simulink model "ssc_refrigeration"  (R2021b)
settings: Solver=VariableStepAuto  StartTime=0.0  StopTime=4000  RelTol=1e-3  AbsTol=1e-3  EnableMultiTasking=on
PreLoadFcn:
  | load r134aPropertyTables
  | 
  | % Refrigerant:
  | initial_pressure = 0.6; % MPa
  | initial_quality = 0.05;
  | 
  | % Environment:
  | environment_temperature = 293; % K
  | natural_convection_coefficient = 20; % W/m^2/K
  | 
  | % Controller:
  | target_temperature = 277; % K
  | temperature_delta = 2; % K
  | 
  | % Compressor:
  | commanded_mass_flow = 0.004; % kg/s
  | controller_time_constant = 20; % s
  | 
  | % Expansion valve:
  | min_throat_area = 0.1; % mm^2
  | max_throat_area = 1.5; % mm^2
  | min_throat_temperature = 270; % K
  | max_throat_temperature = 250; % K
  | 
  | % Heat exchangers:
  | condenser_length = 30; % m
  | evaporator_length = 30; % m
  | fin_area = 1; % m^2
  | fin_convection_coefficient = 150; % W/m^2/K
  | 
  | % Pipes:
  | pipe_diameter = 0.01; % m
  | pipe_thickness = 0.0005; % m
  | 
  | % Refrigerator compartment:
  | interior_surface_area = 4.5; % m^2
  | exterior_surface_area = 6; % m^2
  | foam_thickness = 0.03; % m
  | 
  | % Material properties:
  | copper_density = 8940; % kg/m^3
  | copper_specific_heat = 390; % J/kg/K
  | copper_conductivity = 400; % W/m/K
  | foam_conductivity = 0.03; % W/m/K
libraries: fl_lib x44, nesl_utility x3
CloseFcn:
  | try,close(h1_ssc_refrigeration),end
  | try,close(h2_ssc_refrigeration),end
  | try,close(h3_ssc_refrigeration),end
  | try,close(h4_ssc_refrigeration),end
  | try,close(h5_ssc_refrigeration),end
  | 
  | clear h1_ssc_refrigeration h2_ssc_refrigeration h3_ssc_refrigeration h4_ssc_refrigeration h5_ssc_refrigeration
  | clear simlog_ssc_refrigeration
  | 
  | clear r134aPropertyTables
  | clear initial_pressure initial_quality
  | clear environment_temperature natural_convection_coefficient
  | clear target_temperature temperature_delta
  | clear commanded_mass_flow controller_time_constant
  | clear min_throat_area max_throat_area min_throat_temperature max_throat_temperature
  | clear condenser_length evaporator_length fin_area fin_convection_coefficient
  | clear pipe_diameter pipe_thickness
  | clear interior_surface_area exterior_surface_area foam_thickness
  | clear copper_density copper_specific_heat copper_conductivity foam_conductivity
Description:
  | Two-Phase Fluid Refrigeration
settings Model: Creator=The MathWorks, Inc.  LastModifiedBy=The MathWorks, Inc.
settings SolverCC: AutoScaleAbsTol=off  AlgebraicLoopSolver=TrustRegion
settings DataIOCC: LimitDataPoints=on  MaxDataPoints=10000  SaveFormat=Array  ReturnWorkspaceOutputs=off
settings OptimizationCC: LifeSpan=inf
settings DebuggingCC: AllowSymbolicDim=off  PregeneratedLibrarySubsystemCodeDiagnostic=none  SFUnexpectedBacktrackingDiag=warning  SFNoUnconditionalDefaultTransitionDiag=warning  SFExecutionAtInitializationDiag=none  SFMachineParentedDataDiag=warning  ArithmeticOperatorsInVariantConditions=warning
settings HardwareCC: ProdBitPerPointer=32  ProdBitPerSizeT=32  ProdBitPerPtrDiffT=32  ProdLargestAtomicFloat=None  ProdIntDivRoundTo=Undefined  ProdEndianess=Unspecified  ProdWordSize=32  ProdHWDeviceType=32-bit Generic
settings ModelReferenceCC: PropagateSignalLabelsOutOfModel=off
settings SFSimCC: SimUseLocalCustomCode=off  CustomCodeUndefinedFunction=UseInterfaceOnly
settings RTWCC: RTWUseLocalCustomCode=off
settings CodeAppCC: StateflowObjectComments=on
settings GRTTargetCC: TargetLangStandard=C89/C90 (ANSI)
settings ConfigComp: CovMetricSettings=dw  CovSaveCumulativeToWorkspaceVar=on  CovSaveSingleToWorkspaceVar=on  CovExternalEMLEnable=off  CovSFcnEnable=off
settings SimscapeCC: SimscapeLogType=all  SimscapeLogSimulationStatistics=on  SimscapeLogName=simlog_ssc_refrigeration  SimscapeLogDataHistory=10000

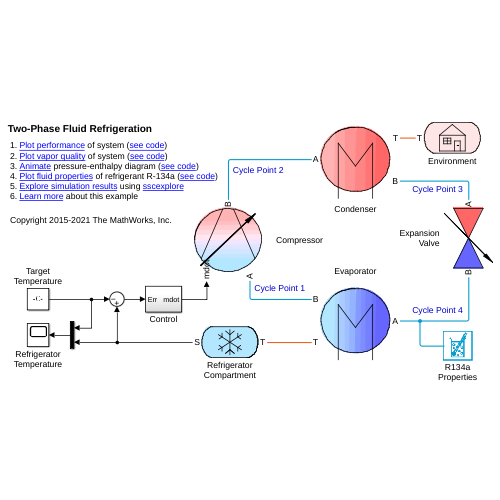
[thumbnail: Simulink's stored preview of the top-level diagram]
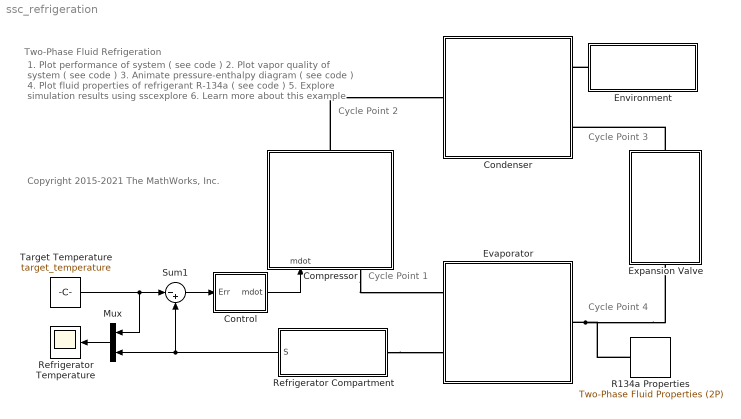
== system ssc_refrigeration ==
  note: Cycle Point 2
  note: Cycle Point 3
  note: 1. Plot performance of system ( see code )
      | 2. Plot vapor quality of system ( see code )
      | 3. Animate pressure-enthalpy diagram ( see code )
      | 4. Plot fluid properties of refrigerant R-134a ( see code )
      | 5. Explore simulation results using sscexplore
      | 6. Learn more about this example
  note: Two-Phase Fluid Refrigeration
  note: Cycle Point 4
  note: Cycle Point 1
  note: Copyright 2015-2021 The MathWorks, Inc.
  Compressor : Subsystem
      mask Display:
      | % Fading color
      | % Center to right
      | patch(sin(0.00*pi:0.05:1.10*pi),cos(0.00*pi:0.05:1.10*pi),[1;0.90;0.94]);
      | patch(sin(0.05*pi:0.05:0.95*pi),cos(0.05*pi:0.05:0.95*pi),[1;0.85;0.88]);
      | patch(sin(0.10*pi:0.05:0.90*pi),cos(0.10*pi:0.05:0.90*pi),[1;0.80;0.82]);
      | patch(sin(0.15*pi:0.05:0.85*pi),cos(0.15*pi:0.05:0.85*pi),[1;0.75;0.76]);
      | patch(sin(0.20*pi:0.05:0.80*pi),cos(0.20*pi:0.05:0.80*pi),[1;0.70;0.70]);
      | % Center to left
      | patch(sin(1.00*pi:0.05:2.00*pi),cos(1.00*pi:0.05:2.00*pi),[0.94;0.90;1]);
      | patch(sin(1.05*pi:0.05:1.95*pi),cos(1.05*pi:0.05:1.95*pi),[0.88;0.90;1]);
      | patch(sin(1.10*pi:0.05:1.90*pi),cos(1.10*pi:0.05:1.90*pi),[0.82;0.90;1]);
      | patch(sin(1.15*pi:0.05:1.85*pi),cos(1.15*pi:0.05:1.85*pi),[0.76;0.90;1]);
      | patch(sin(1.20*pi:0.05:1.80*pi),cos(1.20*pi:0.05:1.80*pi),[0.70;0.90;1]);
      | % Circle
      | plot(sin(0:0.1:2.2*pi),cos(0:0.1:2.2*pi));
      | % Angled lines
      | plot(sin([-0.6*pi/3 3.6*pi/8]),cos([-0.6*pi/3 3.6*pi/8]));
      | plot(sin([-0.6*pi/3 3.6*pi/8]),-cos([-0.6*pi/3 3.6*pi/8]));
      | plot(1.15*sin([-pi/4 3*pi/4]),1.15*cos([-pi/4 3*pi/4]));
      | % Arrow
      | patch([1.15*sin(-pi/4)+0.01;1.15*sin(3*pi/4)+0.01;1.15*sin(3*pi/4)-0.01;1.15*sin(-pi/4)-0.01],[1.15*cos(-pi/4)+0.01;1.15*cos(3*pi/4)+0.01;1.15*cos(3*pi/4)-0.01;1.15*cos(-pi/4)-0.01],[0;0;0])
      | patch([0.8*sin(3*pi/4)+0.05;1.15*sin(3*pi/4)+0.00;1.15*sin(3*pi/4)-0.00;0.8*sin(3*pi/4)-0.05],[0.8*cos(3*pi/4)+0.05;1.15*cos(3*pi/4)+0.00;1.15*cos(3*pi/4)-0.00;0.8*cos(3*pi/4)-0.05],[0;0;0])
      | % Points to set range for plotting area
      | color('white');plot(1.3,1.3);plot(-1.3,-1.3)
      | color('black');
      | 
      | port_label('LConn',1,'A');
      | port_label('RConn',1,'B');
      | port_label('input',1,'mdot');
  Condenser : Subsystem
      mask Display:
      | % Colored patches
      | % Center to right
      | patch(sin(0.0*pi:0.05:1.1*pi),cos(0.0*pi:0.05:1.1*pi),[1;0.58;0.58]);
      | patch(sin(0.1*pi:0.05:0.9*pi),cos(0.1*pi:0.05:0.9*pi),[1;0.64;0.64]);
      | patch(sin(0.2*pi:0.05:0.8*pi),cos(0.2*pi:0.05:0.8*pi),[1;0.70;0.70]);
      | % Center to left
      | patch(sin(1.0*pi:0.05:2.0*pi),cos(1.0*pi:0.05:2.0*pi),[1;0.52;0.52]);
      | patch(sin(1.1*pi:0.05:1.9*pi),cos(1.1*pi:0.05:1.9*pi),[1;0.46;0.46]);
      | patch(sin(1.2*pi:0.05:1.8*pi),cos(1.2*pi:0.05:1.8*pi),[1;0.40;0.40]);
      | % Circle
      | plot(sin(0:0.1:2.2*pi),cos(0:0.1:2.2*pi));
      | % 'M'
      | plot([0.5 0.5],[-1.2 0.5]);
      | plot([-0.5 -0.5],[-1.2 0.5]);
      | plot([0.5 0],[0.5 -0.2]);
      | plot([-0.5 0],[0.5 -0.2]);
      | % Plot points to set plot range
      | color('white');plot(1.3,1.3);plot(-1.3,-1.3)
      | color('black');
      | 
      | port_label('RConn',1,'A');
      | port_label('LConn',1,'T');
      | port_label('LConn',2,'B');
  Control : Subsystem  Tag=CustomStyle
  Environment : Subsystem
      mask Display:
      | % Colored patch
      | patch([sin(0:0.1:1*pi)*0.25+0.4 sin(pi:0.1:2*pi)*0.25-0.4],[cos(0:0.1:1*pi) cos(pi:0.1:2*pi)],[1;0.9;0.9]);
      | % Outer rounded rectangle
      | plot(sin(0:0.1:1*pi)*0.25+0.4,cos(0:0.1:1*pi));
      | plot(sin(pi:0.1:2*pi)*0.25-0.4,cos(pi:0.1:2*pi));
      | plot([-0.4 0.4],[1 1]);
      | plot([-0.4 0.4],[-1 -1]);
      | % House frame
      | plot([-0.3 -0.3],[-0.866,0.866*0.2])
      | plot([0.3 0.3],[-0.866,0.866*0.2])
      | plot([0.3 0],[0.866*0.2, 0.866])
      | plot([-0.3 0],[0.866*0.2, 0.866])
      | plot([-0.3 0.3],[-0.866 -0.866])
      | plot([-0.3 0.3],[0.866 0.866]*0.2)
      | plot([-0.2 -0.04],[0.866 0.866]*0)
      | % Window
      | plot([-0.2 -0.04],[-1 -1]*0.2)
      | plot([-0.2 -0.04],[-1 -1]*0.4)
      | plot([-0.2 -0.2],[0 -0.4])
      | plot([-0.12 -0.12],[0 -0.4])
      | plot([-0.04 -0.04],[0 -0.4])
      | % Door
      | plot([0.05 0.05],[-0.866 -0.2])
      | plot([0.18 0.18],[-0.866 -0.2])
      | plot([0.05 0.18],[-0.2 -0.2])
      | patch([0.12 0.15 0.12 0.15],[-0.5 -0.5 -0.54 -0.54],[0;0;0])
      | % Outer boundary (so plot labels are visible)
      | color('white');plot(0.8660,0.8660);plot(-0.8660,-0.8660)
      | color('black');
      | port_label('LConn',1,'T');
  Evaporator : Subsystem
      mask Display:
      | % Fading color
      | % Center to right
      | patch(sin(0.00*pi:0.05:1.10*pi),cos(0.00*pi:0.05:1.10*pi),[0.58;0.70;1]);
      | patch(sin(0.05*pi:0.05:0.95*pi),cos(0.05*pi:0.05:0.95*pi),[0.63;0.75;1]);
      | patch(sin(0.10*pi:0.05:0.90*pi),cos(0.10*pi:0.05:0.90*pi),[0.66;0.80;1]);
      | patch(sin(0.15*pi:0.05:0.85*pi),cos(0.15*pi:0.05:0.85*pi),[0.69;0.85;1]);
      | patch(sin(0.20*pi:0.05:0.80*pi),cos(0.20*pi:0.05:0.80*pi),[0.70;0.90;1]);
      | % Center to left
      | patch(sin(1.00*pi:0.05:2.00*pi),cos(1.00*pi:0.05:2.00*pi),[0.52;0.60;1]);
      | patch(sin(1.05*pi:0.05:1.95*pi),cos(1.05*pi:0.05:1.95*pi),[0.49;0.55;1]);
      | patch(sin(1.10*pi:0.05:1.90*pi),cos(1.10*pi:0.05:1.90*pi),[0.46;0.50;1]);
      | patch(sin(1.15*pi:0.05:1.85*pi),cos(1.15*pi:0.05:1.85*pi),[0.43;0.45;1]);
      | patch(sin(1.20*pi:0.05:1.80*pi),cos(1.20*pi:0.05:1.80*pi),[0.40;0.40;1]);
      | % Circle
      | plot(sin(0:0.1:2.2*pi),cos(0:0.1:2.2*pi));
      | % 'M'
      | plot([0.5 0.5],[-1.2 0.5]);
      | plot([-0.5 -0.5],[-1.2 0.5]);
      | plot([0.5 0],[0.5 -0.2]);
      | plot([-0.5 0],[0.5 -0.2]);
      | % Plot points to set plotting range
      | color('white');plot(1.3,1.3);plot(-1.3,-1.3)
      | color('black');
      | 
      | port_label('LConn',1,'A');
      | port_label('RConn',1,'B');
      | port_label('RConn',2,'T');
  Expansion Valve : Subsystem
      mask Display:
      | % Colored patches
      | patch([-1 -1 0],[0.5 -0.5 0],[1;0.4;0.4]);
      | patch([1 1 0],[0.5 -0.5 0],[0.4;0.4;1]);
      | % Valve
      | plot([1 1],[0.5 -0.5]);
      | plot([-1 -1],[0.5 -0.5]);
      | plot([-1 1],[0.5 -0.5]);
      | plot([-1 1],[-0.5 0.5]);
      | % Arrow
      | patch([1.15*sin(-pi/4-0.01);1.15*sin(-pi/4+0.01);1*sin(3*pi/4-0.01);1*sin(3*pi/4+0.01)],[1.15*cos(-pi/4-0.01);1.15*cos(-pi/4+0.01);1*cos(3*pi/4-0.01);1*cos(3*pi/4+0.01)],[0;0;0])
      | patch([0.8*sin(3*pi/4+0.07);1.15*sin(3*pi/4+0.00);1.15*sin(3*pi/4-0.00);0.8*sin(3*pi/4-0.07)],[0.8*cos(3*pi/4+0.07);1.15*cos(3*pi/4+0.00);1.15*cos(3*pi/4-0.00);0.8*cos(3*pi/4-0.07)],[0;0;0])
      | % Plot outer points to set plot range
      | color('white'); plot(-1.3,0); plot(1.3,0);
      | color('black');
      | port_label('LConn',1,'A');
      | port_label('RConn',1,'B');
  Mux : Mux  Inputs=2
  R134a Properties : fl_lib/Two-Phase Fluid/Utilities/Two-Phase Fluid Properties (2P)  u_min=r134aPropertyTables.u_min kJ/kg  u_max=r134aPropertyTables.u_max kJ/kg  p_TLU=r134aPropertyTables.p MPa  p_crit=r134aPropertyTables.p_crit MPa  critical_region=foundation.enum.critical_region.clip  p_crit_fraction=0.12  p_atm=0.101325 MPa  q_rev=0.01 Pa  unorm_liq=r134aPropertyTables.liquid.unorm  v_liq=r134aPropertyTables.liquid.v m^3/kg  s_liq=r134aPropertyTables.liquid.s kJ/kg/K  T_liq=r134aPropertyTables.liquid.T K  nu_liq=r134aPropertyTables.liquid.nu mm^2/s  k_liq=r134aPropertyTables.liquid.k W/(m*K)  Pr_liq=r134aPropertyTables.liquid.Pr  u_sat_liq=r134aPropertyTables.liquid.u_sat kJ/kg  unorm_vap=r134aPropertyTables.vapor.unorm  v_vap=r134aPropertyTables.vapor.v m^3/kg  s_vap=r134aPropertyTables.vapor.s kJ/kg/K  T_vap=r134aPropertyTables.vapor.T K  nu_vap=r134aPropertyTables.vapor.nu mm^2/s  k_vap=r134aPropertyTables.vapor.k W/(m*K)  Pr_vap=r134aPropertyTables.vapor.Pr  u_sat_vap=r134aPropertyTables.vapor.u_sat kJ/kg
      settings: SourceProductBaseCode=SS  InternalSimscapePortConfiguration="{\"Bottom\":[],\"Left\":[],\"Right\":[{\"id\":\"A\",\"label\":\"\",\"type\":\"foundation.two_phase_fluid.two_phase_fluid\"}],\"Top\":[]}"
  Refrigerator Compartment : Subsystem
      mask Display:
      | % Color
      | patch([sin(0:0.1:1*pi)*0.25+0.4 sin(pi:0.1:2*pi)*0.25-0.4],[cos(0:0.1:1*pi) cos(pi:0.1:2*pi)],[0.70;0.90;1]);
      | % Outer rounded rectangle
      | plot(sin(pi:0.1:2*pi)*0.25-0.4,cos(pi:0.1:2*pi));
      | plot(sin(0:0.1:1*pi)*0.25+0.4,cos(0:0.1:1*pi));
      | plot(sin(pi:0.1:2*pi)*0.25-0.4,cos(pi:0.1:2*pi));
      | plot([-0.4 0.4],[1 1]);
      | plot([-0.4 0.4],[-1 -1]);
      | % Outer points to set size of plot range
      | color('white');plot(0.8660,0.8660);plot(-0.8660,-0.8660)
      | color('black');
      | % Snowflake
      | plot([0 0],[0.8 -0.8]);
      | plot([0 0.1],[0.5 0.7]);
      | plot([0 -0.1],[0.5 0.7]);
      | plot([0 0.1],[-0.5 -0.7]);
      | plot([0 -0.1],[-0.5 -0.7]);
      | plot(0.3*sin([pi/3 4*pi/3]),1*cos([pi/3 4*pi/3]));
      | plot([0.22*sin(pi/3) 0.25*sin(pi/4)],[0.7*cos(pi/3) 0.84*cos(pi/4)]);
      | plot([0.22*sin(pi/3) 0.25*sin(pi/2)],[0.7*cos(pi/3) 0.325*cos(pi/4)]);
      | plot([0.22*sin(pi/3) 0.25*sin(pi/4)],[-0.7*cos(pi/3) -0.84*cos(pi/4)]);
      | plot([0.22*sin(pi/3) 0.25*sin(pi/2)],[-0.7*cos(pi/3) -0.325*cos(pi/4)]);
      | plot(-0.3*sin([pi/3 4*pi/3]),1*cos([pi/3 4*pi/3]));
      | plot([-0.22*sin(pi/3) -0.25*sin(pi/4)],[0.7*cos(pi/3) 0.84*cos(pi/4)]);
      | plot([-0.22*sin(pi/3) -0.25*sin(pi/2)],[0.7*cos(pi/3) 0.325*cos(pi/4)]);
      | plot([-0.22*sin(pi/3) -0.25*sin(pi/4)],[-0.7*cos(pi/3) -0.84*cos(pi/4)]);
      | plot([-0.22*sin(pi/3) -0.25*sin(pi/2)],[-0.7*cos(pi/3) -0.325*cos(pi/4)]);
      | plot([0 0.1],[-0.5 -0.7]);
      | plot([0 -0.1],[-0.5 -0.7]);
      | % Labels
      | port_label('LConn',1,'T');
      | port_label('output',1,'S');
  Refrigerator Temperature : Scope
  Sum1 : Sum  Inputs=|-+
  Target Temperature : Constant  Value=target_temperature
  wires:
  Target Temperature/1 -> Mux/1, Sum1/1
  Refrigerator Compartment/1(S) -> Mux/2, Sum1/2
  Sum1/1 -> Control/1(Err)
  Control/1(mdot) -> Compressor/1(mdot)
  Mux/1 -> Refrigerator Temperature/1
  connections:
  Evaporator/LConn1 -- R134a Properties/RConn1 -- Expansion Valve/RConn1
  Expansion Valve/LConn1 -- Condenser/LConn2
  Compressor/RConn1 -- Condenser/RConn1
  Environment/LConn1 -- Condenser/LConn1
  Compressor/LConn1 -- Evaporator/RConn1
  Refrigerator Compartment/LConn1 -- Evaporator/RConn2

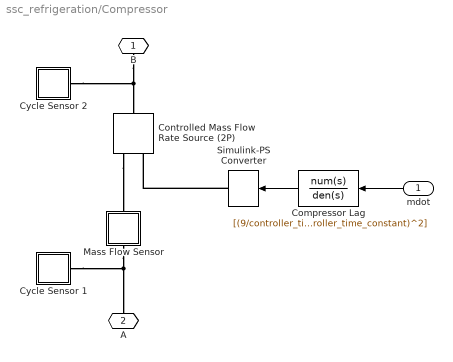
== system ssc_refrigeration/Compressor ==
  mdot : Inport
  Compressor Lag : TransferFcn  Numerator=[(9/controller_time_constant)^2]  Denominator=[1, 2*(9/controller_time_constant), (9/controller_time_constant)^2]
  Controlled Mass Flow Rate Source (2P) : fl_lib/Two-Phase Fluid/Sources/Controlled Mass Flow Rate Source (2P)  power_spec=1  area_A=pi*pipe_diameter^2/4 m^2  area_B=pi*pipe_diameter^2/4 m^2
      settings: SourceProductBaseCode=SS  InternalSimscapePortConfiguration="{\"Bottom\":[],\"Left\":[{\"id\":\"A\",\"label\":\"A\",\"type\":\"foundation.two_phase_fluid.two_phase_fluid\"},{\"id\":\"M\",\"label\":\"M\",\"type\":\"input\"}],\"Right\":[{\"id\":\"B\",\"label\":\"B\",\"type\":\"foundation.two_phase_fluid.two_phase_fluid\"}],\"Top\":[]}"
  Cycle Sensor 1 : Subsystem
  Cycle Sensor 2 : Subsystem
  Mass Flow Sensor : Subsystem
  Simulink-PS Converter : nesl_utility/Simulink-PS Converter  PhysicalDomain=network_engine_domain  SubClassName=ps_input  LeftPortType=input  RightPortType=output  PseudoPeriodic=off  Frequencies=[]  NoiseDistribution=none  NoiseParameters=[]  Unit=kg/s  AffineConversion=off  FilteringAndDerivatives=zero  SimscapeFilterOrder=1  InputFilterTimeConstant=0.001  UdotUserProvided=1
      settings: SourceProductBaseCode=PW,SS
  B : PMIOPort  Side=Right
  A : PMIOPort  Port=2  Side=Left
  wires:
  Compressor Lag/1 -> Simulink-PS Converter/1
  mdot/1 -> Compressor Lag/1
  connections:
  Cycle Sensor 2/LConn1 -- Controlled Mass Flow Rate Source (2P)/RConn1 -- B/RConn1
  Mass Flow Sensor/LConn1 -- A/RConn1 -- Cycle Sensor 1/LConn1
  Controlled Mass Flow Rate Source (2P)/LConn1 -- Mass Flow Sensor/RConn1
  Simulink-PS Converter/RConn1 -- Controlled Mass Flow Rate Source (2P)/LConn2

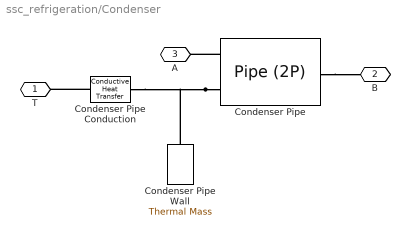
== system ssc_refrigeration/Condenser ==
  Condenser Pipe Wall : fl_lib/Thermal/Thermal Elements/Thermal Mass  mass=pi*pipe_diameter*condenser_length*pipe_thickness*copper_density kg  sp_heat=copper_specific_heat J/kg/K  T_specify=on  T_priority=High  T=environment_temperature K  T_nominal_specify=off  T_nominal_unit=K  T_nominal_value=1  Q_specify=off  Q_priority=None  Q=0 W  Q_nominal_specify=off  Q_nominal_unit=W  Q_nominal_value=1
  Condenser Pipe : fl_lib/Two-Phase Fluid/Elements/Pipe (2P)  length=condenser_length m  area=pi*pipe_diameter^2/4 m^2  Dh=pipe_diameter m  length_add=0.1*condenser_length m  roughness=1.5e-5 m  Re_lam=2e+3  Re_tur=4e+3  shape_factor=64  Nu_lam=3.66  inertia=0  energy_spec=foundation.enum.energy_spec.quality  p_init=initial_pressure MPa  T_init=293.15 K  x_init=initial_quality  alpha_init=0.5  h_init=1500 kJ/kg  u_init=1500 kJ/kg  mdot_init=0 kg/s  time_constant=0.1 s
      settings: SourceProductBaseCode=SS  InternalSimscapePortConfiguration="{\"Bottom\":[],\"Left\":[{\"id\":\"A\",\"label\":\"A\",\"type\":\"foundation.two_phase_fluid.two_phase_fluid\"},{\"id\":\"H\",\"label\":\"H\",\"type\":\"foundation.thermal.thermal\"}],\"Right\":[{\"id\":\"B\",\"label\":\"B\",\"type\":\"foundation.two_phase_fluid.two_phase_fluid\"}],\"Top\":[]}"
  Condenser Pipe Conduction : fl_lib/Thermal/Thermal Elements/Conductive Heat Transfer  area=pi*pipe_diameter*condenser_length m^2  thickness=pipe_thickness m  th_cond=copper_conductivity W/(m*K)  T_specify=off  T_priority=None  T=0 K  T_nominal_specify=off  T_nominal_unit=K  T_nominal_value=1  Q_specify=off  Q_priority=None  Q=0 W  Q_nominal_specify=off  Q_nominal_unit=W  Q_nominal_value=1
  T : PMIOPort  Side=Left
  B : PMIOPort  Port=2  Side=Left
  A : PMIOPort  Port=3  Side=Right
  connections:
  Condenser Pipe/LConn2 -- Condenser Pipe Conduction/LConn1 -- Condenser Pipe Wall/LConn1
  Condenser Pipe/LConn1 -- A/RConn1
  Condenser Pipe/RConn1 -- B/RConn1
  Condenser Pipe Conduction/RConn1 -- T/RConn1

== system ssc_refrigeration/Control ==
  Err : Inport
  Mass Flow Rate : Gain  Gain=commanded_mass_flow
  Relay : Relay  OnSwitchValue=temperature_delta  OffSwitchValue=-temperature_delta
  mdot : Outport  VectorParamsAs1DForOutWhenUnconnected=off
  wires:
  Err/1 -> Relay/1
  Relay/1 -> Mass Flow Rate/1
  Mass Flow Rate/1 -> mdot/1

== system ssc_refrigeration/Environment ==
  Condenser Convection : fl_lib/Thermal/Thermal Elements/Convective Heat Transfer  area=fin_area m^2  heat_tr_coeff=fin_convection_coefficient W/(m^2 * K)  T_specify=off  T_priority=None  T=0 K  T_nominal_specify=off  T_nominal_unit=K  T_nominal_value=1  Q_specify=off  Q_priority=None  Q=0 W  Q_nominal_specify=off  Q_nominal_unit=W  Q_nominal_value=1
  Environment Temperature : fl_lib/Thermal/Thermal Sources/Temperature Source  temperature=environment_temperature K
  Solver Configuration : nesl_utility/Solver Configuration  PhysicalDomain=network_engine_domain  SubClassName=solver  LeftPortType=input  RightPortType=generic  Tones=[]  Harmonics=[]  SimulateNoise=off  Profile=off  UseLocalSampling=off  EnableSwitchedLinearOptims=on  FrequencyDomain=off  UseCCode=off  RelTol=0.001  AbsTol=1e-06  MinStep=1e-09  ToWorkspace=off  RevertToSquareIcSolve=off  NumHomotopyIterations=100  PhasorMode=off  PhasorModeNumHarmonics=1  DoDC=off  ResidualTolerance=1e-9  UseLocalSolver=off  LocalSolverChoice=NE_BACKWARD_EULER_ADVANCER  LocalSolverSampleTime=1  DoFixedCost=off  MaxNonlinIter=3  MaxModeIter=2  ComputeImpulses=off  ImpulseIterations=2  LinearAlgebra=auto  EquationFormulation=NE_TIME_EF  DelaysMemoryBudget=1024  AutomaticFiltering=on  FilteringTimeConstant=0.001  PartitionStorageMethod=AS_NEEDED  PartitionMemoryBudget=1024  PartitionMethod=FAST
      settings: SourceProductBaseCode=PW,SS
  T : PMIOPort  Side=Left
  connections:
  Condenser Convection/RConn1 -- Solver Configuration/RConn1 -- Environment Temperature/LConn1
  Condenser Convection/LConn1 -- T/RConn1

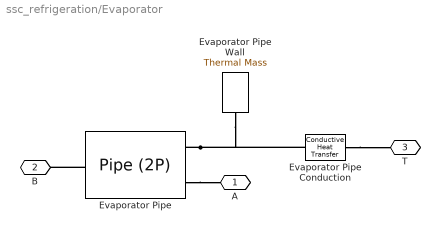
== system ssc_refrigeration/Evaporator ==
  Evaporator Pipe Wall : fl_lib/Thermal/Thermal Elements/Thermal Mass  mass=pi*pipe_diameter*evaporator_length*pipe_thickness*copper_density kg  sp_heat=copper_specific_heat J/kg/K  T_specify=on  T_priority=High  T=target_temperature K  T_nominal_specify=off  T_nominal_unit=K  T_nominal_value=1  Q_specify=off  Q_priority=None  Q=0 W  Q_nominal_specify=off  Q_nominal_unit=W  Q_nominal_value=1
  Evaporator Pipe : fl_lib/Two-Phase Fluid/Elements/Pipe (2P)  length=evaporator_length m  area=pi*pipe_diameter^2/4 m^2  Dh=pipe_diameter m  length_add=0.1*evaporator_length m  roughness=1.5e-5 m  Re_lam=2e+3  Re_tur=4e+3  shape_factor=64  Nu_lam=3.66  inertia=0  energy_spec=foundation.enum.energy_spec.quality  p_init=initial_pressure MPa  T_init=293.15 K  x_init=initial_quality  alpha_init=0.5  h_init=1500 kJ/kg  u_init=1500 kJ/kg  mdot_init=0 kg/s  time_constant=0.1 s
      settings: SourceProductBaseCode=SS  InternalSimscapePortConfiguration="{\"Bottom\":[],\"Left\":[{\"id\":\"A\",\"label\":\"A\",\"type\":\"foundation.two_phase_fluid.two_phase_fluid\"},{\"id\":\"H\",\"label\":\"H\",\"type\":\"foundation.thermal.thermal\"}],\"Right\":[{\"id\":\"B\",\"label\":\"B\",\"type\":\"foundation.two_phase_fluid.two_phase_fluid\"}],\"Top\":[]}"
  Evaporator Pipe Conduction : fl_lib/Thermal/Thermal Elements/Conductive Heat Transfer  area=pi*pipe_diameter*evaporator_length m^2  thickness=pipe_thickness m  th_cond=copper_conductivity W/(m*K)  T_specify=off  T_priority=None  T=0 K  T_nominal_specify=off  T_nominal_unit=K  T_nominal_value=1  Q_specify=off  Q_priority=None  Q=0 W  Q_nominal_specify=off  Q_nominal_unit=W  Q_nominal_value=1
  A : PMIOPort  Side=Left
  B : PMIOPort  Port=2  Side=Right
  T : PMIOPort  Port=3  Side=Right
  connections:
  Evaporator Pipe/LConn2 -- Evaporator Pipe Conduction/LConn1 -- Evaporator Pipe Wall/LConn1
  Evaporator Pipe/LConn1 -- A/RConn1
  Evaporator Pipe Conduction/RConn1 -- T/RConn1
  Evaporator Pipe/RConn1 -- B/RConn1

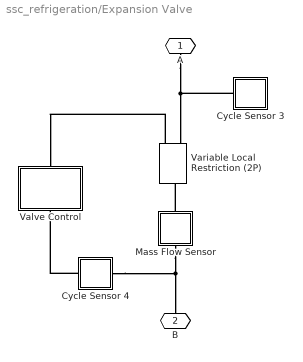
== system ssc_refrigeration/Expansion Valve ==
  Cycle Sensor 3 : Subsystem
  Cycle Sensor 4 : Subsystem
  Mass Flow Sensor : Subsystem
  Valve Control : Subsystem
  Variable Local Restriction (2P) : fl_lib/Two-Phase Fluid/Elements/Variable Local Restriction (2P)  min_area=min_throat_area mm^2  max_area=max_throat_area mm^2  area=pi*pipe_diameter^2/4 m^2  Cd=0.7  B_lam=0.999
      settings: SourceProductBaseCode=SS  InternalSimscapePortConfiguration="{\"Bottom\":[],\"Left\":[{\"id\":\"A\",\"label\":\"A\",\"type\":\"foundation.two_phase_fluid.two_phase_fluid\"},{\"id\":\"area_in\",\"label\":\"AR\",\"type\":\"input\"}],\"Right\":[{\"id\":\"B\",\"label\":\"B\",\"type\":\"foundation.two_phase_fluid.two_phase_fluid\"}],\"Top\":[]}"
  A : PMIOPort  Side=Left
  B : PMIOPort  Port=2  Side=Right
  connections:
  Cycle Sensor 4/LConn1 -- B/RConn1 -- Mass Flow Sensor/RConn1
  Cycle Sensor 3/LConn1 -- A/RConn1 -- Variable Local Restriction (2P)/LConn1
  Mass Flow Sensor/LConn1 -- Variable Local Restriction (2P)/RConn1
  Cycle Sensor 4/RConn1 -- Valve Control/RConn1
  Variable Local Restriction (2P)/LConn2 -- Valve Control/LConn1

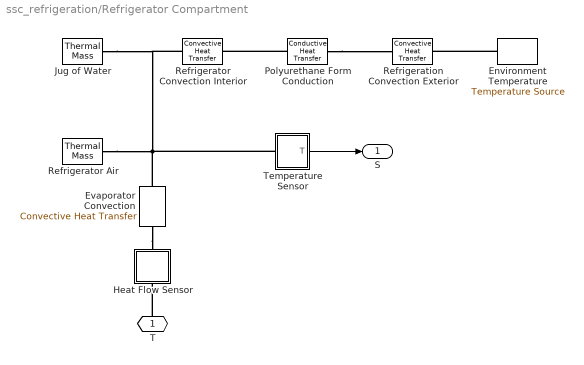
== system ssc_refrigeration/Refrigerator Compartment ==
  Environment Temperature : fl_lib/Thermal/Thermal Sources/Temperature Source  temperature=environment_temperature K
  Evaporator Convection : fl_lib/Thermal/Thermal Elements/Convective Heat Transfer  area=interior_surface_area m^2  heat_tr_coeff=natural_convection_coefficient W/(m^2 * K)  T_specify=off  T_priority=None  T=0 K  T_nominal_specify=off  T_nominal_unit=K  T_nominal_value=1  Q_specify=off  Q_priority=None  Q=0 W  Q_nominal_specify=off  Q_nominal_unit=W  Q_nominal_value=1
  Heat Flow Sensor : Subsystem
  Jug of Water : fl_lib/Thermal/Thermal Elements/Thermal Mass  mass=3.8 kg  sp_heat=4187 J/kg/K  T_specify=on  T_priority=High  T=target_temperature K  T_nominal_specify=off  T_nominal_unit=K  T_nominal_value=1  Q_specify=off  Q_priority=None  Q=0 W  Q_nominal_specify=off  Q_nominal_unit=W  Q_nominal_value=1
  Polyurethane Form Conduction : fl_lib/Thermal/Thermal Elements/Conductive Heat Transfer  area=interior_surface_area m^2  thickness=foam_thickness m  th_cond=foam_conductivity W/(m*K)  T_specify=off  T_priority=None  T=0 K  T_nominal_specify=off  T_nominal_unit=K  T_nominal_value=1  Q_specify=off  Q_priority=None  Q=0 W  Q_nominal_specify=off  Q_nominal_unit=W  Q_nominal_value=1
  Refrigeration Convection Exterior : fl_lib/Thermal/Thermal Elements/Convective Heat Transfer  area=exterior_surface_area m^2  heat_tr_coeff=natural_convection_coefficient W/(m^2 * K)  T_specify=off  T_priority=None  T=0 K  T_nominal_specify=off  T_nominal_unit=K  T_nominal_value=1  Q_specify=off  Q_priority=None  Q=0 W  Q_nominal_specify=off  Q_nominal_unit=W  Q_nominal_value=1
  Refrigerator Air : fl_lib/Thermal/Thermal Elements/Thermal Mass  mass=1 kg  sp_heat=1012 J/kg/K  T_specify=on  T_priority=High  T=target_temperature K  T_nominal_specify=off  T_nominal_unit=K  T_nominal_value=1  Q_specify=off  Q_priority=None  Q=0 W  Q_nominal_specify=off  Q_nominal_unit=W  Q_nominal_value=1
  Refrigerator Convection Interior : fl_lib/Thermal/Thermal Elements/Convective Heat Transfer  area=interior_surface_area m^2  heat_tr_coeff=natural_convection_coefficient W/(m^2 * K)  T_specify=off  T_priority=None  T=0 K  T_nominal_specify=off  T_nominal_unit=K  T_nominal_value=1  Q_specify=off  Q_priority=None  Q=0 W  Q_nominal_specify=off  Q_nominal_unit=W  Q_nominal_value=1
  Temperature Sensor : Subsystem
  T : PMIOPort  Side=Left
  S : Outport  VectorParamsAs1DForOutWhenUnconnected=off
  wires:
  Temperature Sensor/1(T) -> S/1
  connections:
  Refrigerator Convection Interior/LConn1 -- Jug of Water/LConn1 -- Evaporator Convection/RConn1 -- Refrigerator Air/LConn1 -- Temperature Sensor/LConn1
  Environment Temperature/LConn1 -- Refrigeration Convection Exterior/RConn1
  Evaporator Convection/LConn1 -- Heat Flow Sensor/RConn1
  Polyurethane Form Conduction/LConn1 -- Refrigerator Convection Interior/RConn1
  T/RConn1 -- Heat Flow Sensor/LConn1
  Polyurethane Form Conduction/RConn1 -- Refrigeration Convection Exterior/LConn1

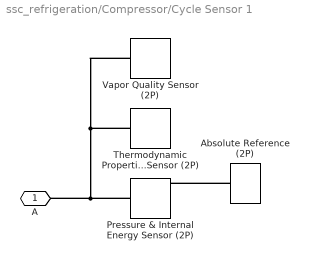
== system ssc_refrigeration/Compressor/Cycle Sensor 1 ==
  Absolute Reference (2P) : fl_lib/Two-Phase Fluid/Elements/Absolute Reference (2P)
      settings: SourceProductBaseCode=SS
  Pressure & Internal Energy Sensor (2P) : fl_lib/Two-Phase Fluid/Sensors/Pressure & Internal Energy Sensor (2P)
      settings: SourceProductBaseCode=SS  InternalSimscapePortConfiguration="{\"Bottom\":[],\"Left\":[{\"id\":\"A\",\"label\":\"A\",\"type\":\"foundation.two_phase_fluid.two_phase_fluid\"}],\"Right\":[{\"id\":\"B\",\"label\":\"B\",\"type\":\"foundation.two_phase_fluid.two_phase_fluid\"},{\"id\":\"P\",\"label\":\"P\",\"type\":\"output\"},{\"id\":\"U\",\"label\":\"U\",\"type\":\"output\"}],\"Top\":[]}"
  Thermodynamic Properties Sensor (2P) : fl_lib/Two-Phase Fluid/Sensors/Thermodynamic Properties Sensor (2P)
      settings: SourceProductBaseCode=SS  InternalSimscapePortConfiguration="{\"Bottom\":[],\"Left\":[{\"id\":\"A\",\"label\":\"A\",\"type\":\"foundation.two_phase_fluid.two_phase_fluid\"}],\"Right\":[{\"id\":\"T\",\"label\":\"T\",\"type\":\"output\"},{\"id\":\"H\",\"label\":\"h\",\"type\":\"output\"},{\"id\":\"V\",\"label\":\"v\",\"type\":\"output\"},{\"id\":\"S\",\"label\":\"s\",\"type\":\"output\"}],\"Top\":[]}"
  Vapor Quality Sensor (2P) : fl_lib/Two-Phase Fluid/Sensors/Vapor Quality Sensor (2P)  vapor_fraction_spec=foundation.enum.vapor_fraction_spec.quality
      settings: SourceProductBaseCode=SS  InternalSimscapePortConfiguration="{\"Bottom\":[],\"Left\":[{\"id\":\"A\",\"label\":\"A\",\"type\":\"foundation.two_phase_fluid.two_phase_fluid\"}],\"Right\":[{\"id\":\"X\",\"label\":\"X\",\"type\":\"output\"}],\"Top\":[]}"
  A : PMIOPort  Side=Left
  connections:
  Thermodynamic Properties Sensor (2P)/LConn1 -- Vapor Quality Sensor (2P)/LConn1 -- A/RConn1 -- Pressure & Internal Energy Sensor (2P)/LConn1
  Absolute Reference (2P)/LConn1 -- Pressure & Internal Energy Sensor (2P)/RConn1

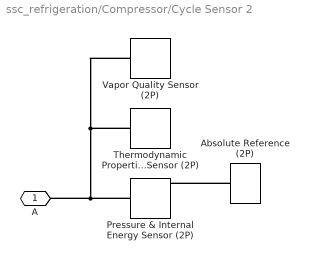
== system ssc_refrigeration/Compressor/Cycle Sensor 2 ==
  Absolute Reference (2P) : fl_lib/Two-Phase Fluid/Elements/Absolute Reference (2P)
      settings: SourceProductBaseCode=SS
  Pressure & Internal Energy Sensor (2P) : fl_lib/Two-Phase Fluid/Sensors/Pressure & Internal Energy Sensor (2P)
      settings: SourceProductBaseCode=SS  InternalSimscapePortConfiguration="{\"Bottom\":[],\"Left\":[{\"id\":\"A\",\"label\":\"A\",\"type\":\"foundation.two_phase_fluid.two_phase_fluid\"}],\"Right\":[{\"id\":\"B\",\"label\":\"B\",\"type\":\"foundation.two_phase_fluid.two_phase_fluid\"},{\"id\":\"P\",\"label\":\"P\",\"type\":\"output\"},{\"id\":\"U\",\"label\":\"U\",\"type\":\"output\"}],\"Top\":[]}"
  Thermodynamic Properties Sensor (2P) : fl_lib/Two-Phase Fluid/Sensors/Thermodynamic Properties Sensor (2P)
      settings: SourceProductBaseCode=SS  InternalSimscapePortConfiguration="{\"Bottom\":[],\"Left\":[{\"id\":\"A\",\"label\":\"A\",\"type\":\"foundation.two_phase_fluid.two_phase_fluid\"}],\"Right\":[{\"id\":\"T\",\"label\":\"T\",\"type\":\"output\"},{\"id\":\"H\",\"label\":\"h\",\"type\":\"output\"},{\"id\":\"V\",\"label\":\"v\",\"type\":\"output\"},{\"id\":\"S\",\"label\":\"s\",\"type\":\"output\"}],\"Top\":[]}"
  Vapor Quality Sensor (2P) : fl_lib/Two-Phase Fluid/Sensors/Vapor Quality Sensor (2P)  vapor_fraction_spec=foundation.enum.vapor_fraction_spec.quality
      settings: SourceProductBaseCode=SS  InternalSimscapePortConfiguration="{\"Bottom\":[],\"Left\":[{\"id\":\"A\",\"label\":\"A\",\"type\":\"foundation.two_phase_fluid.two_phase_fluid\"}],\"Right\":[{\"id\":\"X\",\"label\":\"X\",\"type\":\"output\"}],\"Top\":[]}"
  A : PMIOPort  Side=Left
  connections:
  Thermodynamic Properties Sensor (2P)/LConn1 -- Vapor Quality Sensor (2P)/LConn1 -- A/RConn1 -- Pressure & Internal Energy Sensor (2P)/LConn1
  Absolute Reference (2P)/LConn1 -- Pressure & Internal Energy Sensor (2P)/RConn1

== system ssc_refrigeration/Compressor/Mass Flow Sensor ==
  Mass & Energy Flow Rate Sensor (2P) : fl_lib/Two-Phase Fluid/Sensors/Mass & Energy Flow Rate Sensor (2P)
      settings: SourceProductBaseCode=SS  InternalSimscapePortConfiguration="{\"Bottom\":[],\"Left\":[{\"id\":\"A\",\"label\":\"A\",\"type\":\"foundation.two_phase_fluid.two_phase_fluid\"}],\"Right\":[{\"id\":\"B\",\"label\":\"B\",\"type\":\"foundation.two_phase_fluid.two_phase_fluid\"},{\"id\":\"M\",\"label\":\"M\",\"type\":\"output\"},{\"id\":\"PHI\",\"label\":\"Phi\",\"type\":\"output\"}],\"Top\":[]}"
  B : PMIOPort  Side=Right
  A : PMIOPort  Port=2  Side=Left
  connections:
  Mass & Energy Flow Rate Sensor (2P)/LConn1 -- A/RConn1
  Mass & Energy Flow Rate Sensor (2P)/RConn1 -- B/RConn1

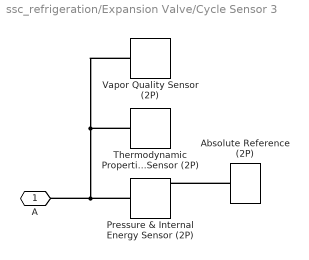
== system ssc_refrigeration/Expansion Valve/Cycle Sensor 3 ==
  Absolute Reference (2P) : fl_lib/Two-Phase Fluid/Elements/Absolute Reference (2P)
      settings: SourceProductBaseCode=SS
  Pressure & Internal Energy Sensor (2P) : fl_lib/Two-Phase Fluid/Sensors/Pressure & Internal Energy Sensor (2P)
      settings: SourceProductBaseCode=SS  InternalSimscapePortConfiguration="{\"Bottom\":[],\"Left\":[{\"id\":\"A\",\"label\":\"A\",\"type\":\"foundation.two_phase_fluid.two_phase_fluid\"}],\"Right\":[{\"id\":\"B\",\"label\":\"B\",\"type\":\"foundation.two_phase_fluid.two_phase_fluid\"},{\"id\":\"P\",\"label\":\"P\",\"type\":\"output\"},{\"id\":\"U\",\"label\":\"U\",\"type\":\"output\"}],\"Top\":[]}"
  Thermodynamic Properties Sensor (2P) : fl_lib/Two-Phase Fluid/Sensors/Thermodynamic Properties Sensor (2P)
      settings: SourceProductBaseCode=SS  InternalSimscapePortConfiguration="{\"Bottom\":[],\"Left\":[{\"id\":\"A\",\"label\":\"A\",\"type\":\"foundation.two_phase_fluid.two_phase_fluid\"}],\"Right\":[{\"id\":\"T\",\"label\":\"T\",\"type\":\"output\"},{\"id\":\"H\",\"label\":\"h\",\"type\":\"output\"},{\"id\":\"V\",\"label\":\"v\",\"type\":\"output\"},{\"id\":\"S\",\"label\":\"s\",\"type\":\"output\"}],\"Top\":[]}"
  Vapor Quality Sensor (2P) : fl_lib/Two-Phase Fluid/Sensors/Vapor Quality Sensor (2P)  vapor_fraction_spec=foundation.enum.vapor_fraction_spec.quality
      settings: SourceProductBaseCode=SS  InternalSimscapePortConfiguration="{\"Bottom\":[],\"Left\":[{\"id\":\"A\",\"label\":\"A\",\"type\":\"foundation.two_phase_fluid.two_phase_fluid\"}],\"Right\":[{\"id\":\"X\",\"label\":\"X\",\"type\":\"output\"}],\"Top\":[]}"
  A : PMIOPort  Side=Left
  connections:
  Thermodynamic Properties Sensor (2P)/LConn1 -- Vapor Quality Sensor (2P)/LConn1 -- A/RConn1 -- Pressure & Internal Energy Sensor (2P)/LConn1
  Absolute Reference (2P)/LConn1 -- Pressure & Internal Energy Sensor (2P)/RConn1

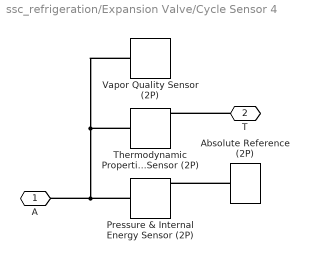
== system ssc_refrigeration/Expansion Valve/Cycle Sensor 4 ==
  Absolute Reference (2P) : fl_lib/Two-Phase Fluid/Elements/Absolute Reference (2P)
      settings: SourceProductBaseCode=SS
  Pressure & Internal Energy Sensor (2P) : fl_lib/Two-Phase Fluid/Sensors/Pressure & Internal Energy Sensor (2P)
      settings: SourceProductBaseCode=SS  InternalSimscapePortConfiguration="{\"Bottom\":[],\"Left\":[{\"id\":\"A\",\"label\":\"A\",\"type\":\"foundation.two_phase_fluid.two_phase_fluid\"}],\"Right\":[{\"id\":\"B\",\"label\":\"B\",\"type\":\"foundation.two_phase_fluid.two_phase_fluid\"},{\"id\":\"P\",\"label\":\"P\",\"type\":\"output\"},{\"id\":\"U\",\"label\":\"U\",\"type\":\"output\"}],\"Top\":[]}"
  Thermodynamic Properties Sensor (2P) : fl_lib/Two-Phase Fluid/Sensors/Thermodynamic Properties Sensor (2P)
      settings: SourceProductBaseCode=SS  InternalSimscapePortConfiguration="{\"Bottom\":[],\"Left\":[{\"id\":\"A\",\"label\":\"A\",\"type\":\"foundation.two_phase_fluid.two_phase_fluid\"}],\"Right\":[{\"id\":\"T\",\"label\":\"T\",\"type\":\"output\"},{\"id\":\"H\",\"label\":\"h\",\"type\":\"output\"},{\"id\":\"V\",\"label\":\"v\",\"type\":\"output\"},{\"id\":\"S\",\"label\":\"s\",\"type\":\"output\"}],\"Top\":[]}"
  Vapor Quality Sensor (2P) : fl_lib/Two-Phase Fluid/Sensors/Vapor Quality Sensor (2P)  vapor_fraction_spec=foundation.enum.vapor_fraction_spec.quality
      settings: SourceProductBaseCode=SS  InternalSimscapePortConfiguration="{\"Bottom\":[],\"Left\":[{\"id\":\"A\",\"label\":\"A\",\"type\":\"foundation.two_phase_fluid.two_phase_fluid\"}],\"Right\":[{\"id\":\"X\",\"label\":\"X\",\"type\":\"output\"}],\"Top\":[]}"
  A : PMIOPort  Side=Left
  T : PMIOPort  Port=2  Side=Right
  connections:
  Thermodynamic Properties Sensor (2P)/LConn1 -- Vapor Quality Sensor (2P)/LConn1 -- A/RConn1 -- Pressure & Internal Energy Sensor (2P)/LConn1
  Absolute Reference (2P)/LConn1 -- Pressure & Internal Energy Sensor (2P)/RConn1
  T/RConn1 -- Thermodynamic Properties Sensor (2P)/RConn1

== system ssc_refrigeration/Expansion Valve/Mass Flow Sensor ==
  Mass & Energy Flow Rate Sensor (2P) : fl_lib/Two-Phase Fluid/Sensors/Mass & Energy Flow Rate Sensor (2P)
      settings: SourceProductBaseCode=SS  InternalSimscapePortConfiguration="{\"Bottom\":[],\"Left\":[{\"id\":\"A\",\"label\":\"A\",\"type\":\"foundation.two_phase_fluid.two_phase_fluid\"}],\"Right\":[{\"id\":\"B\",\"label\":\"B\",\"type\":\"foundation.two_phase_fluid.two_phase_fluid\"},{\"id\":\"M\",\"label\":\"M\",\"type\":\"output\"},{\"id\":\"PHI\",\"label\":\"Phi\",\"type\":\"output\"}],\"Top\":[]}"
  B : PMIOPort  Side=Right
  A : PMIOPort  Port=2  Side=Left
  connections:
  Mass & Energy Flow Rate Sensor (2P)/LConn1 -- A/RConn1
  Mass & Energy Flow Rate Sensor (2P)/RConn1 -- B/RConn1

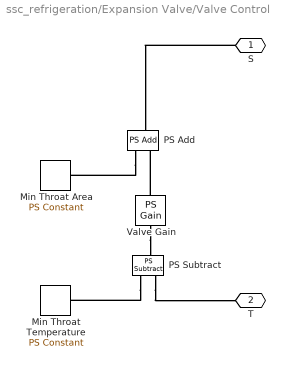
== system ssc_refrigeration/Expansion Valve/Valve Control ==
  Min Throat Area : fl_lib/Physical Signals/Sources/PS Constant  constant=min_throat_area mm^2
  Min Throat Temperature : fl_lib/Physical Signals/Sources/PS Constant  constant=min_throat_temperature K
  PS Add : fl_lib/Physical Signals/Functions/PS Add
  PS Subtract : fl_lib/Physical Signals/Functions/PS Subtract
  Valve Gain : fl_lib/Physical Signals/Functions/PS Gain  gain=(max_throat_area - min_throat_area)/(max_throat_temperature - min_throat_temperature) mm^2/K
  S : PMIOPort  Side=Left
  T : PMIOPort  Port=2  Side=Right
  connections:
  PS Subtract/LConn1 -- T/RConn1
  PS Add/LConn1 -- Min Throat Area/RConn1
  PS Subtract/LConn2 -- Min Throat Temperature/RConn1
  Valve Gain/LConn1 -- PS Subtract/RConn1
  Valve Gain/RConn1 -- PS Add/LConn2
  S/RConn1 -- PS Add/RConn1

== system ssc_refrigeration/Refrigerator Compartment/Heat Flow Sensor ==
  Heat Flow Rate Sensor : fl_lib/Thermal/Thermal Sensors/Heat Flow Rate Sensor
      settings: SourceProductBaseCode=SS
  B : PMIOPort  Side=Right
  A : PMIOPort  Port=2  Side=Left
  connections:
  Heat Flow Rate Sensor/LConn1 -- A/RConn1
  Heat Flow Rate Sensor/RConn2 -- B/RConn1

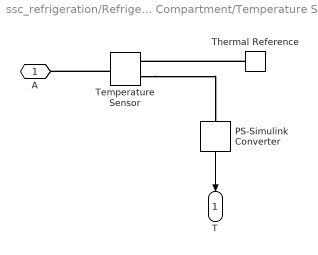
== system ssc_refrigeration/Refrigerator Compartment/Temperature Sensor ==
  PS-Simulink Converter : nesl_utility/PS-Simulink Converter  PhysicalDomain=network_engine_domain  SubClassName=ps_output  LeftPortType=input  RightPortType=output  PseudoPeriodic=off  Frequencies=[]  Unit=K  AffineConversion=off
      settings: SourceProductBaseCode=PW,SS
  Temperature Sensor : fl_lib/Thermal/Thermal Sensors/Temperature Sensor
  Thermal Reference : fl_lib/Thermal/Thermal Elements/Thermal Reference
  A : PMIOPort  Side=Left
  T : Outport  VectorParamsAs1DForOutWhenUnconnected=off
  wires:
  PS-Simulink Converter/1 -> T/1
  connections:
  Temperature Sensor/LConn1 -- A/RConn1
  Thermal Reference/LConn1 -- Temperature Sensor/RConn1
  Temperature Sensor/RConn2 -- PS-Simulink Converter/LConn1
